simulink model "piCtrl"  (R2023b)
settings: Solver=FixedStepDiscrete  StartTime=0.0  StopTime=10.0  FixedStep=Ts  RelTol=1e-3  EnableMultiTasking=on
undefined symbols (not defined in the file): Ki, Kp, Ts
settings Model: RequirementInfo={} %GIDa_8782a213_6690_4762_8fd4_78a65de31043  Creator=jrivitus  LastModifiedBy=student
settings SolverCC: MaxConsecutiveZCs=25  AlgebraicLoopSolver=TrustRegion
settings DataIOCC: DSMLogging=off  ReturnWorkspaceOutputs=off
settings OptimizationCC: DefaultParameterBehavior=Inlined  ExpressionDepthLimit=2147483647  InitFltsAndDblsToZero=on  LifeSpan=1  EfficientTunableParamExpr=on
settings DebuggingCC: UnderspecifiedInitializationDetection=Classic  MergeDetectMultiDrivingBlocksExec=none  ParameterPrecisionLossMsg=none  FcnCallInpInsideContextMsg=warning  UnconnectedInputMsg=warning  UnconnectedOutputMsg=warning  UnconnectedLineMsg=warning  AllowSymbolicDim=off  StateNameClashWarn=warning  PregeneratedLibrarySubsystemCodeDiagnostic=none  SFUnexpectedBacktrackingDiag=warning  SFNoUnconditionalDefaultTransitionDiag=warning  SFExecutionAtInitializationDiag=none  ArithmeticOperatorsInVariantConditions=warning
settings HardwareCC: ProdLongLongMode=on
settings ModelReferenceCC: UpdateModelReferenceTargets=IfOutOfDate  EnableRefExpFcnMdlSchedulingChecks=on  PropagateSignalLabelsOutOfModel=off
settings SFSimCC: SimUseLocalCustomCode=off  MATLABDynamicMemAlloc=off
settings RTWCC: Description=Embedded Coder  SystemTargetFile=ert.tlc  TemplateMakefile=ert_default_tmf  RTWUseLocalCustomCode=off  DLArmComputeVersion=19.05
settings CodeAppCC: IgnoreCustomStorageClasses=off  StateflowObjectComments=on
settings ERTTargetCC: MultiwordLength=2048  GenerateSampleERTMain=on  InlinedParameterPlacement=NonHierarchical  ERTCustomFileTemplate=example_file_process.tlc  ConvertIfToSwitch=off  SuppressUnreachableDefaultCases=off
settings ConfigComp: CovMetricSettings=dcmwe  CovHTMLOptions=-sRT=1 -sVT=0 -aTS=1 -bRG=1 -bTC=1 -hTR=0 -nFC=0 -nFD=1 -scm=1 -bcm=1 -xEv=0 -xEM=0  CovSaveCumulativeToWorkspaceVar=on  CovExternalEMLEnable=off  CovSFcnEnable=off  DVTestSuiteOptimization=CombinedObjectives (Nonlinear Extended)  DVIgnoreExistTestSatisfied=off

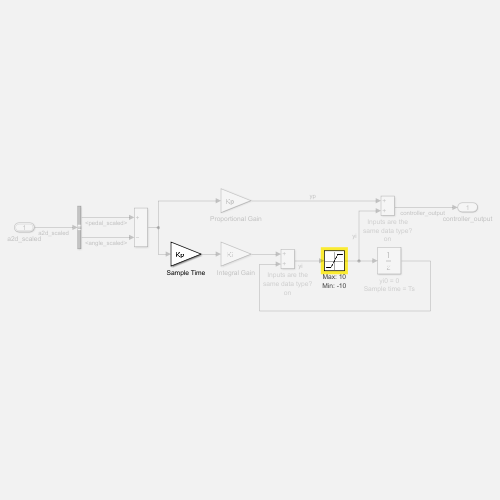
[thumbnail: Simulink's stored preview of the top-level diagram]
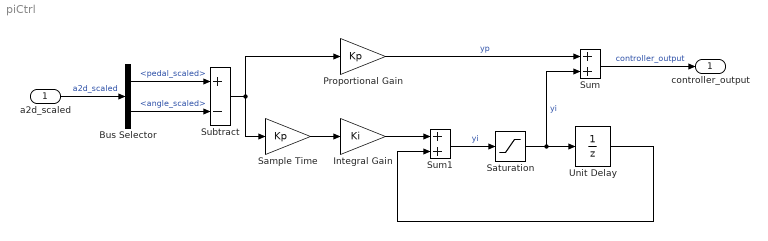
== system piCtrl ==
  a2d_scaled : Inport  OutDataTypeStr=Bus: a2d_scaled_bus  PortDimensions=1  SampleTime=Ts
  Bus Selector : BusSelector  OutputSignals=pedal_scaled,angle_scaled
  Integral Gain : Gain  Gain=Ki  SaturateOnIntegerOverflow=on  OutDataTypeStr=Inherit: Same as input  ParamDataTypeStr=Inherit: Same as input
  Proportional Gain : Gain  Gain=Kp  SaturateOnIntegerOverflow=on  OutDataTypeStr=Inherit: Same as input  ParamDataTypeStr=Inherit: Same as input
  Sample Time : Gain  Gain=Kp  SaturateOnIntegerOverflow=on  OutDataTypeStr=Inherit: Same as input  ParamDataTypeStr=Inherit: Same as input
  Saturation : Saturate  UpperLimit=10  LowerLimit=-10
      settings: AttributesFormatString=|
      | Max: %<UpperLimit>
      | Min: %<LowerLimit>
  Subtract : Sum  Inputs=+-
  Sum : Sum  InputSameDT=on  SaturateOnIntegerOverflow=on  OutDataTypeStr=Inherit: Same as first input
      settings: AttributesFormatString=|
      | Inputs are the
      | same data type?
      | %<InputSameDT>
  Sum1 : Sum  InputSameDT=on  SaturateOnIntegerOverflow=on  OutDataTypeStr=Inherit: Same as first input
      settings: AttributesFormatString=|
      | Inputs are the
      | same data type?
      | %<InputSameDT>
  Unit Delay : UnitDelay  SampleTime=Ts  HasFrameUpgradeWarning=on
      settings: AttributesFormatString=yi0 = %<X0>\nSample time = %<SampleTime>
  controller_output : Outport  OutDataTypeStr=double  PortDimensions=1  SampleTime=Ts  VectorParamsAs1DForOutWhenUnconnected=off
  wires:
  a2d_scaled/1 -> Bus Selector/1  "a2d_scaled"
  Subtract/1 -> Sample Time/1, Proportional Gain/1
  Bus Selector/2 -> Subtract/2  "<angle_scaled>"
  Bus Selector/1 -> Subtract/1  "<pedal_scaled>"
  Proportional Gain/1 -> Sum/1  "yp"
  Integral Gain/1 -> Sum1/1
  Sample Time/1 -> Integral Gain/1
  Unit Delay/1 -> Sum1/2
  Sum/1 -> controller_output/1  "controller_output"
  Sum1/1 -> Saturation/1  "yi"
  Saturation/1 -> Sum/2, Unit Delay/1  "yi"
